simulink model "Regulator_Solver"  (R2016b)
settings: Solver=ode23tb  StartTime=0.0  StopTime=10.0  MaxStep=0.01  RelTol=1e-3
settings Model: Creator=rfdej  LastModifiedBy=Niels
settings SolverCC: ZeroCrossAlgorithm=Adaptive

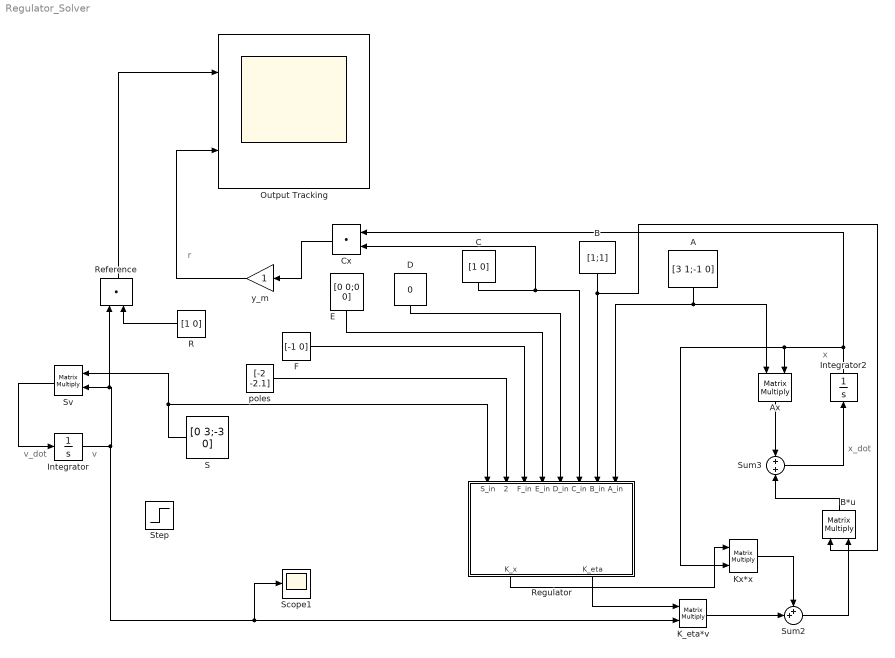
== system Regulator_Solver ==
  note: x_dot
  note: x
  note: r
  note: v
  note: v_dot
  A : Constant  Value=[3 1;-1 0]
  Ax : Product  Multiplication=Matrix(*)
  B : Constant  Value=[1;1]  VectorParams1D=off
  B*u : Product  Multiplication=Matrix(*)
  C : Constant  Value=[1 0]  VectorParams1D=off
  Cx : DotProduct  InputSameDT=on  OutDataTypeStr=Inherit: Inherit via internal rule
  D : Constant  Value=0
  E : Constant  Value=[0 0;0 0]
  F : Constant  Value=[-1 0]  VectorParams1D=off
  Integrator : Integrator  InitialCondition=[1;0]
  Integrator2 : Integrator  InitialCondition=[1 1]
  K_eta*v : Product  Multiplication=Matrix(*)
  Kx*x : Product  Multiplication=Matrix(*)
  Output Tracking : Scope  NumInputPorts=2
  R : Constant  Value=[1 0]
  Reference : DotProduct  InputSameDT=on  OutDataTypeStr=Inherit: Inherit via internal rule
  Regulator : Subsystem
  S : Constant  Value=[0 3;-3 0]
  Scope1 : Scope
  Step : Step  SampleTime=0
  Sum2 : Sum  Inputs=++|
  Sum3 : Sum  Inputs=+|+
  Sv : Product  Inputs=**  Multiplication=Matrix(*)
  poles : Constant  Value=[-2 -2.1]
  y_m : Gain
  wires:
  S/1 -> Sv/1, Regulator/1(S_in)
  Sv/1 -> Integrator/1
  R/1 -> Reference/2
  Integrator/1 -> K_eta*v/2, Scope1/1, Sv/2, Reference/1
  C/1 -> Regulator/6(C_in), Cx/2
  B/1 -> B*u/1, Regulator/7(B_in)
  A/1 -> Regulator/8(A_in), Ax/1
  Integrator2/1 -> Cx/1, Ax/2, Kx*x/2
  Kx*x/1 -> Sum2/1
  K_eta*v/1 -> Sum2/2
  B*u/1 -> Sum3/2
  Ax/1 -> Sum3/1
  Sum3/1 -> Integrator2/1
  Sum2/1 -> B*u/2
  Reference/1 -> Output Tracking/1
  poles/1 -> Regulator/2(poles_in)
  D/1 -> Regulator/5(D_in)
  F/1 -> Regulator/3(F_in)
  E/1 -> Regulator/4(E_in)
  Regulator/2(K_eta) -> K_eta*v/1
  Regulator/1(K_x) -> Kx*x/1
  Cx/1 -> y_m/1
  y_m/1 -> Output Tracking/2

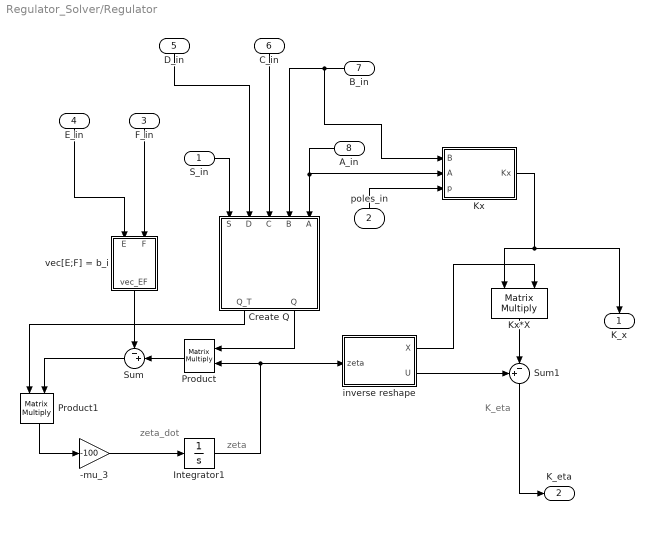
== system Regulator_Solver/Regulator ==
  note: K_eta
  note: zeta_dot
  note: zeta
  S_in : Inport
  poles_in : Inport  Port=2
  F_in : Inport  Port=3
  E_in : Inport  Port=4
  D_in : Inport  Port=5
  C_in : Inport  Port=6
  B_in : Inport  Port=7
  A_in : Inport  Port=8
  -mu_3 : Gain  Gain=-100
  Create Q : MATLAB Function  TreatAsAtomicUnit=on
  Integrator1 : Integrator  InitialCondition=[1;1;1;1;1;1]
  Kx : MATLAB Function  TreatAsAtomicUnit=on
  Kx*X : Product  Inputs=**  Multiplication=Matrix(*)
  Product : Product  Multiplication=Matrix(*)
  Product1 : Product  Multiplication=Matrix(*)
  Sum : Sum  Inputs=-+|
  Sum1 : Sum  Inputs=+-|
  inverse reshape : MATLAB Function  TreatAsAtomicUnit=on
  "vec[E;F] = b_i   " : MATLAB Function  TreatAsAtomicUnit=on
  K_x : Outport
  K_eta : Outport  Port=2
  wires:
  inverse reshape/1(X) -> Kx*X/2
  inverse reshape/2(U) -> Sum1/1
  F_in/1 -> "vec[E;F] = b_i   "/2(F)
  Create Q/2(Q) -> Product/1
  Product1/1 -> -mu_3/1
  Sum1/1 -> K_eta/1
  Sum/1 -> Product1/2
  Create Q/1(Q_T) -> Product1/1
  Kx*X/1 -> Sum1/2
  poles_in/1 -> Kx/3(p)
  Integrator1/1 -> Product/2, inverse reshape/1(zeta)
  -mu_3/1 -> Integrator1/1
  Kx/1(Kx) -> Kx*X/1, K_x/1
  S_in/1 -> Create Q/1(S)
  A_in/1 -> Create Q/5(A), Kx/2(A)
  C_in/1 -> Create Q/3(C)
  B_in/1 -> Kx/1(B), Create Q/4(B)
  D_in/1 -> Create Q/2(D)
  E_in/1 -> "vec[E;F] = b_i   "/1(E)
  "vec[E;F] = b_i   "/1(vec_EF) -> Sum/1
  Product/1 -> Sum/2

== matlab function Regulator_Solver/Regulator/vec[E;F] = b_i    ==
  data: E input; vec_EF output; F input
function vec_EF = fcn(E,F)


vec_EF = reshape([E;F],6,1);
end

== matlab function Regulator_Solver/Regulator/Create Q ==
  data: Q_T output; Q output; S input; D input; C input; B input; A input
function [Q_T,Q]= fcn(S,D,C,B,A)

I_ni_id = eye(2);
I_ni = [I_ni_id [0;0];0 0 0];
I_q = eye(2);
sysmatrix = [A B;C D];

Q = kron(S.',I_ni)-kron(I_q,sysmatrix);
Q_T = Q.';
end

== matlab function Regulator_Solver/Regulator/inverse reshape ==
  data: zeta input; X output; U output
function [X,U] = fcn(zeta)

tmp = reshape(zeta,3,2);
X = tmp(1:2,1:2);
U = tmp(3,:);
end

== matlab function Regulator_Solver/Regulator/Kx ==
  data: B input; A input; Kx output; p input
function Kx = fcn(B,A,p)

coder.extrinsic('place')
Kx = zeros(1,2);
Kx = place(A,-B,p);
